simulink model "direct_form_rea"  (R2020b)
settings: Solver=VariableStepAuto  StartTime=0.0  StopTime=10.0  RelTol=1e-3
settings Model: Creator=Arvind Hishikar  LastModifiedBy=Arvind Hishikar
settings DataIOCC: SaveOutput=off  SaveTime=off

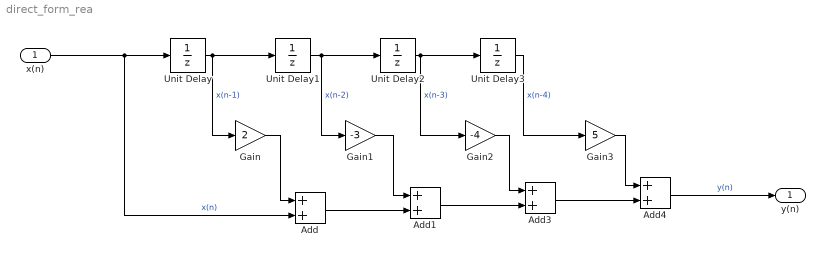
== system direct_form_rea ==
  x(n) : Inport  OutDataTypeStr=double  PortDimensions=1  SampleTime=[0,1]
  Add{,1,3..4} (4 alike) : Sum
  Gain : Gain  Gain=2
  Gain1 : Gain  Gain=-3
  Gain2 : Gain  Gain=-4
  Gain3 : Gain  Gain=5
  Unit Delay{,1..3} (4 alike) : UnitDelay  SampleTime=-1  HasFrameUpgradeWarning=on
  y(n) : Outport  OutDataTypeStr=double  PortDimensions=1  SampleTime=[0,1]
  wires:
  Gain3/1 -> Add4/1
  x(n)/1 -> Add/2, Unit Delay/1  "x(n)"
  Unit Delay/1 -> Gain/1, Unit Delay1/1  "x(n-1)"
  Unit Delay2/1 -> Gain2/1, Unit Delay3/1  "x(n-3)"
  Unit Delay1/1 -> Gain1/1, Unit Delay2/1  "x(n-2)"
  Unit Delay3/1 -> Gain3/1  "x(n-4)"
  Gain1/1 -> Add1/1
  Add/1 -> Add1/2
  Gain2/1 -> Add3/1
  Gain/1 -> Add/1
  Add1/1 -> Add3/2
  Add3/1 -> Add4/2
  Add4/1 -> y(n)/1  "y(n)"
